simulink model "Main"  (R2021a)
settings: Solver=ode4  StartTime=0.0  StopTime=param.taskDuration  FixedStep=0.02  RelTol=1e-3
InitFcn:
  | Init
StopFcn:
  | StopSim
values from neighbouring files (symbols this model uses):
  kuka = kuka.InitializeJacobian(kuka, KukaInitialJoint, vrepInstance, 1)    [Init.m]
  ur = ur.InitializeJacobian(ur, URInitialJoint, vrepInstance, 1)    [Init.m]
undefined symbols (not defined in the file or in its folder): DiscIntNeverNeededParam, param
settings Model: EnablePacing=on  Creator=dell  LastModifiedBy=dell

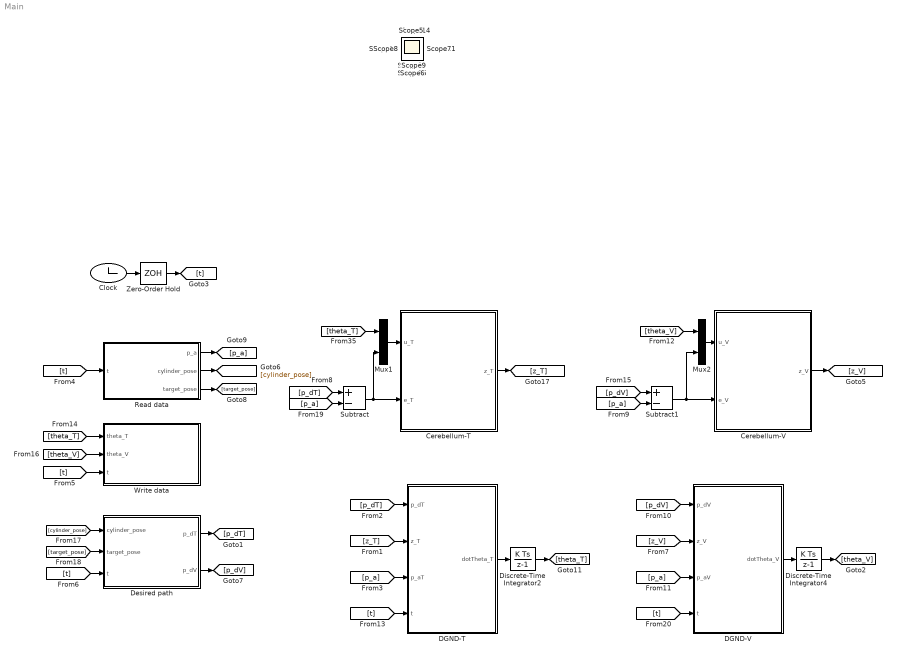
== system Main ==
  Cerebellum-T : MATLAB Function  TreatAsAtomicUnit=on
  Cerebellum-V : MATLAB Function  TreatAsAtomicUnit=on
  Clock : Clock
  DGND-T : MATLAB Function  TreatAsAtomicUnit=on
  DGND-V : MATLAB Function  TreatAsAtomicUnit=on
  Desired path : MATLAB Function  TreatAsAtomicUnit=on
  Discrete-Time Integrator2 : DiscreteIntegrator  InitialCondition=ur.theta(:,1)  SampleTime=-1  OutDataTypeStr=double  ICPrevOutput=DiscIntNeverNeededParam  ICPrevScaledInput=DiscIntNeverNeededParam
  Discrete-Time Integrator4 : DiscreteIntegrator  InitialCondition=kuka.theta(:,1)  SampleTime=-1  OutDataTypeStr=double  ICPrevOutput=DiscIntNeverNeededParam  ICPrevScaledInput=DiscIntNeverNeededParam
  Mux1 : Mux  Inputs=2
  Mux2 : Mux  Inputs=2
  Read data : MATLAB Function  TreatAsAtomicUnit=on
  Subtract : Sum  Inputs=+-
  Subtract1 : Sum  Inputs=+-
  Write data : MATLAB Function  TreatAsAtomicUnit=on
  Zero-Order Hold : ZeroOrderHold  SampleTime=param.samplingGap
  Scope{,1..15} (16 alike) : Scope
  wires:
  Clock/1 -> Zero-Order Hold/1
  Zero-Order Hold/1 -> [t]
  [t] -> Read data/1(t)
  [theta_T] -> Write data/1(theta_T)
  Discrete-Time Integrator2/1 -> [theta_T]
  Read data/1(p_a) -> [p_a]
  [p_dT] -> Subtract/1
  [p_a] -> Subtract/2
  Mux1/1 -> Cerebellum-T/1(u_T)
  Cerebellum-T/1(z_T) -> [z_T]
  [theta_T] -> Mux1/1
  Subtract/1 -> Mux1/2, Cerebellum-T/2(e_T)
  Desired path/1(p_dT) -> [p_dT]
  [z_T] -> DGND-T/2(z_T)
  [p_dT] -> DGND-T/1(p_dT)
  [p_a] -> DGND-T/3(p_aT)
  DGND-T/1(dotTheta_T) -> Discrete-Time Integrator2/1
  DGND-V/1(dotTheta_V) -> Discrete-Time Integrator4/1
  [p_a] -> DGND-V/3(p_aV)
  [p_dV] -> DGND-V/1(p_dV)
  [z_V] -> DGND-V/2(z_V)
  Subtract1/1 -> Cerebellum-V/2(e_V), Mux2/2
  [theta_V] -> Mux2/1
  Cerebellum-V/1(z_V) -> [z_V]
  Mux2/1 -> Cerebellum-V/1(u_V)
  [p_a] -> Subtract1/2
  [p_dV] -> Subtract1/1
  Discrete-Time Integrator4/1 -> [theta_V]
  Read data/2(cylinder_pose) -> [cylinder_pose]
  Desired path/2(p_dV) -> [p_dV]
  [theta_V] -> Write data/2(theta_V)
  Read data/3(target_pose) -> [target_pose]
  [cylinder_pose] -> Desired path/1(cylinder_pose)
  [target_pose] -> Desired path/2(target_pose)
  [t] -> Write data/3(t)
  [t] -> Desired path/3(t)
  [t] -> DGND-T/4(t)
  [t] -> DGND-V/4(t)

== matlab function Main/Read data ==
  data: t input; p_a output; cylinder_pose output; target_pose output
function [p_a, cylinder_pose, target_pose]  = VREPRead(t)

coder.extrinsic('VrepRead');

p_a = zeros(6,1);
cylinder_pose = zeros(6,1);
target_pose = zeros(6,1);

output = double(VrepRead(t));

p_a = output(1:6);
cylinder_pose = output(7:12);
target_pose = output(13:18);

== matlab function Main/Write data ==
  data: theta_T input; theta_V input; t input
function VREPWrite(theta_T, theta_V, t)

coder.extrinsic('VrepWrite');
% To keep the robot stationary when Simulink begins to execute
% if t>0
    VrepWrite(theta_T, theta_V, t)
% end

== matlab function Main/DGND-T ==
  data: p_dT input; z_T input; p_aT input; dotTheta_T output; t input
function dotTheta_T    = DGND_T(p_dT, z_T, p_aT, t)
coder.extrinsic('DGND_T');
dotTheta_T = zeros(6,1);

output = double(DGND_T(p_dT, z_T, p_aT, t));
dotTheta_T = output(1:6);

== matlab function Main/Desired path ==
  data: p_dT output; p_dV output; cylinder_pose input; target_pose input; t input
function [p_dT, p_dV] = Path_Gnrt(cylinder_pose, target_pose, t)
%#codegen

coder.extrinsic('PathGnrt');
p_dT = zeros(6,1);
p_dV = zeros(6,1);
output = double(PathGnrt(cylinder_pose, target_pose, t));
p_dT = output(1:6);
p_dV = output(7:12);

== matlab function Main/Cerebellum-V ==
  data: u_V input; z_V output; e_V input
function z_V  = Cereb_Net(u_V, e_V)
coder.extrinsic('CerebNet_V');

z_V = zeros(6,1);
output = double(CerebNet_V(u_V, e_V));
z_V = output;

== matlab function Main/DGND-V ==
  data: p_dV input; z_V input; p_aV input; dotTheta_V output; t input
function dotTheta_V    = DGND_V(p_dV, z_V, p_aV, t)
coder.extrinsic('DGND_V');
dotTheta_V = zeros(7,1);
dotJHat_V = zeros(7,7);

output = double(DGND_V(p_dV, z_V, p_aV, t));
dotTheta_V = output(1:7);

== matlab function Main/Cerebellum-T ==
  data: u_T input; z_T output; e_T input
function z_T  = Cereb_Net(u_T, e_T)
coder.extrinsic('CerebNet_T');

z_T = zeros(6,1);
output = double(CerebNet_T(u_T, e_T));
z_T = output;
